simulink model "ch7example25"  (Simulink 5.0)
settings: Solver=ode45  StartTime=0.0  StopTime=1000.0  MaxStep=1e-4  RelTol=1e-3
undefined symbols (not defined in the file): Fs
libraries: commutil2 x3, simulink x3, dspsnks4 x2, commdigbbndpm2 x1, commrandsrc2 x1, commseqgen2 x1
settings Model: LastModifiedBy=shaoyubin

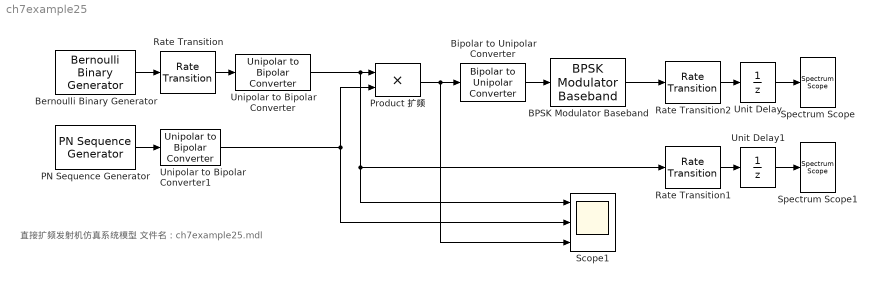
== system ch7example25 ==
  note: 直接扩频发射机仿真系统模型
      | 文件名：ch7example25.mdl
  BPSK Modulator Baseband : commdigbbndpm2/BPSK Modulator Baseband  Ph=0  numSamp=1
  Bernoulli Binary Generator : commrandsrc2/Bernoulli Binary Generator  P=0.5  seed=61  Ts=1/100  frameBased=off  sampPerFrame=1  orient=off
  Bipolar to Unipolar Converter : commutil2/Bipolar to Unipolar Converter  M=2  polarity=Positive
  PN Sequence Generator : commseqgen2/PN Sequence Generator  poly=[1 0 0 0 0 1 1]  ini_sta=[0 0 0 0 0 1]  shift=0  Ts=1/2000  frameBased=off  sampPerFrame=1  reset=off
  Product 扩频 : Product  SaturateOnIntegerOverflow=on
  Rate Transition : simulink/Signal Attributes/Rate Transition  DataIntegrity=on  DeterministicTransfer=on  TransitionType=Slow to fast  InitCond=0
  Rate Transition1 : simulink/Signal Attributes/Rate Transition  DataIntegrity=on  DeterministicTransfer=on  TransitionType=Slow to fast  InitCond=0
  Rate Transition2 : simulink/Signal Attributes/Rate Transition  DataIntegrity=on  DeterministicTransfer=on  TransitionType=Slow to fast  InitCond=0
  Scope1 : Scope  NumInputPorts=3
      settings: TickLabels=off  TimeRange=0.1  YMin=-5~-5~-5  YMax=5~5~5
  Spectrum Scope : dspsnks4/Spectrum Scope  ScopeProperties=on  Domain=Frequency  HorizSpan=1  UseBuffer=on  BufferSize=1024  Overlap=512  inpFftLenInherit=on  FFTlength=1024  numAvg=500  DisplayProperties=off  AxisGrid=on  Memory=off  FrameNumber=on  AxisLegend=off  AxisZoom=off  OpenScopeAtSimStart=on  OpenScopeImmediately=off  FigPos=[232 258 560 420]  AxisProperties=off  XUnits=Hertz  XRange=[-Fs/2...Fs/2]  InheritXIncr=on  XIncr=1  XLabel=Samples  YUnits=dB  YLabel=Magnitude, dB  LineProperties=off  LineMarkers=|None  LineColors=|[1 0 0]
      settings: YMin=-48.9282442585022  YMax=23.2359531120033
  Spectrum Scope1 : dspsnks4/Spectrum Scope  ScopeProperties=on  Domain=Frequency  HorizSpan=1  UseBuffer=on  BufferSize=1024  Overlap=512  inpFftLenInherit=on  FFTlength=1024  numAvg=500  DisplayProperties=off  AxisGrid=on  Memory=off  FrameNumber=off  AxisLegend=off  AxisZoom=off  OpenScopeAtSimStart=on  OpenScopeImmediately=off  FigPos=[232 258 560 420]  AxisProperties=off  XUnits=Hertz  XRange=[-Fs/2...Fs/2]  InheritXIncr=on  XIncr=1  XLabel=Samples  YUnits=dB  YLabel=Magnitude, dB  LineProperties=off  LineMarkers=|None  LineColors=|[1 0 0]
      settings: YMin=-48.9282442585022  YMax=23.2359531120033
  Unipolar to Bipolar Converter : commutil2/Unipolar to Bipolar Converter  M=2  polarity=Positive
  Unipolar to Bipolar Converter1 : commutil2/Unipolar to Bipolar Converter  M=2  polarity=Positive
  Unit Delay : UnitDelay  SampleTime=1/8000
  Unit Delay1 : UnitDelay  SampleTime=1/8000
  wires:
  Bernoulli Binary Generator/1 -> Rate Transition/1
  PN Sequence Generator/1 -> Unipolar to Bipolar Converter1/1
  Product 扩频/1 -> Bipolar to Unipolar Converter/1, Scope1/3
  Rate Transition/1 -> Unipolar to Bipolar Converter/1
  Unit Delay/1 -> Spectrum Scope/1
  Rate Transition2/1 -> Unit Delay/1
  Unipolar to Bipolar Converter/1 -> Product 扩频/1, Rate Transition1/1, Scope1/1
  Bipolar to Unipolar Converter/1 -> BPSK Modulator Baseband/1
  Unipolar to Bipolar Converter1/1 -> Product 扩频/2, Scope1/2
  BPSK Modulator Baseband/1 -> Rate Transition2/1
  Unit Delay1/1 -> Spectrum Scope1/1
  Rate Transition1/1 -> Unit Delay1/1
